simulink model "chap6_1sim"  (Simulink 3.00)
settings: Solver=ode45  SolverMode=SingleTasking  StartTime=0.0  StopTime=3  FixedStep=0.001  RelTol=1e-5  AbsTol=1e-5
settings Model: LastModifiedBy=liu

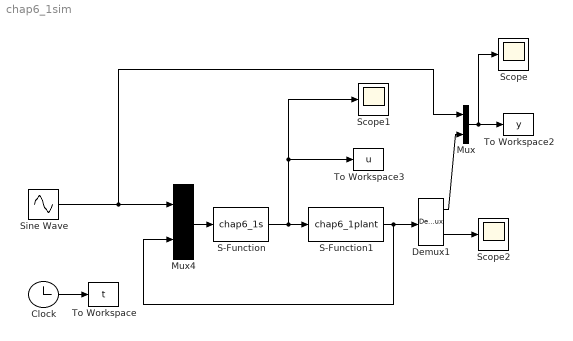
== system chap6_1sim ==
  Clock : Clock
  Demux1 : Demux  Outputs=2
  Mux : Mux  Inputs=2
  Mux4 : Mux  Inputs=2
      settings: DisplayOption=none
  S-Function : S-Function  FunctionName=chap6_1s  PortCounts=[]  SFunctionModules=''
  S-Function1 : S-Function  FunctionName=chap6_1plant  PortCounts=[]  SFunctionModules=''
  Scope : Scope
      settings: TimeRange=auto  YMin=-1  YMax=1  SaveToWorkspace=off  SaveName=ScopeData
  Scope1 : Scope
      settings: TimeRange=auto  YMin=-125  YMax=125  SaveToWorkspace=off  SaveName=ScopeData
  Scope2 : Scope
      settings: TimeRange=auto  YMin=-8  YMax=8  SaveToWorkspace=off  SaveName=ScopeData
  Sine Wave : Sin  Amplitude=1  Frequency=3*2*pi  Phase=0  SampleTime=0
  To Workspace : ToWorkspace  VariableName=t  SampleTime=-1  SaveFormat=Matrix
  To Workspace2 : ToWorkspace  VariableName=y  SampleTime=-1  SaveFormat=Matrix
  To Workspace3 : ToWorkspace  VariableName=u  SampleTime=-1  SaveFormat=Matrix
  wires:
  Mux4/1 -> S-Function/1
  Mux/1 -> To Workspace2/1, Scope/1
  S-Function/1 -> S-Function1/1, To Workspace3/1, Scope1/1
  Demux1/1 -> Mux/2
  Demux1/2 -> Scope2/1
  S-Function1/1 -> Demux1/1, Mux4/2
  Sine Wave/1 -> Mux/1, Mux4/1
  Clock/1 -> To Workspace/1
